simulink model "MIL_MarleyOS_Powertrain"  (R2026a)
settings: Solver=VariableStepAuto  StopTime=10
settings Model: Creator=UsuarioPC  LastModifiedBy=UsuarioPC
settings DataIOCC: ExternalInput=CommunicationDataset  LoadExternalInput=on

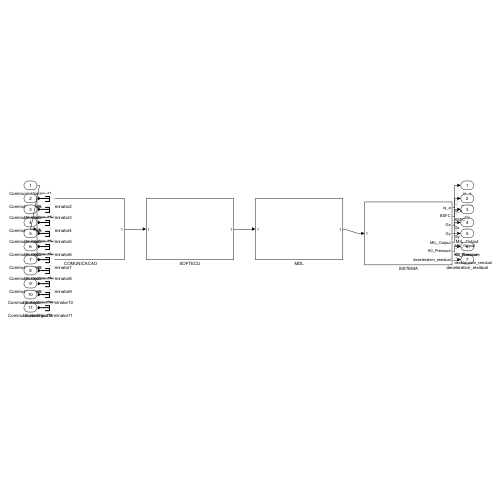
[thumbnail: Simulink's stored preview of the top-level diagram]
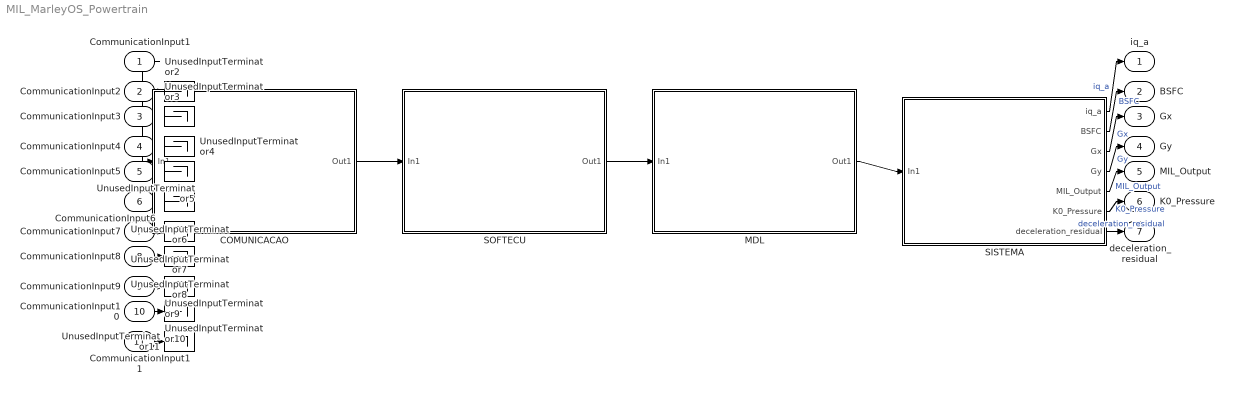
== system MIL_MarleyOS_Powertrain ==
  CommunicationInput1 : Inport
  CommunicationInput2 : Inport  Port=2
  CommunicationInput3 : Inport  Port=3
  CommunicationInput4 : Inport  Port=4
  CommunicationInput5 : Inport  Port=5
  CommunicationInput6 : Inport  Port=6
  CommunicationInput7 : Inport  Port=7
  CommunicationInput8 : Inport  Port=8
  CommunicationInput9 : Inport  Port=9
  CommunicationInput10 : Inport  Port=10
  CommunicationInput11 : Inport  Port=11
  COMUNICACAO : Subsystem
  MDL : Subsystem
  SISTEMA : Subsystem
  SOFTECU : Subsystem
  UnusedInputTerminator{2..11} (10 alike) : Terminator
  iq_a : Outport
  BSFC : Outport  Port=2
  Gx : Outport  Port=3
  Gy : Outport  Port=4
  MIL_Output : Outport  Port=5
  K0_Pressure : Outport  Port=6
  deceleration_residual : Outport  Port=7
  wires:
  CommunicationInput1/1 -> COMUNICACAO/1(In1)
  CommunicationInput2/1 -> UnusedInputTerminator2/1
  CommunicationInput3/1 -> UnusedInputTerminator3/1
  CommunicationInput4/1 -> UnusedInputTerminator4/1
  CommunicationInput5/1 -> UnusedInputTerminator5/1
  CommunicationInput6/1 -> UnusedInputTerminator6/1
  CommunicationInput7/1 -> UnusedInputTerminator7/1
  CommunicationInput8/1 -> UnusedInputTerminator8/1
  CommunicationInput9/1 -> UnusedInputTerminator9/1
  CommunicationInput10/1 -> UnusedInputTerminator10/1
  CommunicationInput11/1 -> UnusedInputTerminator11/1
  COMUNICACAO/1(Out1) -> SOFTECU/1(In1)
  SOFTECU/1(Out1) -> MDL/1(In1)
  MDL/1(Out1) -> SISTEMA/1(In1)
  SISTEMA/1(iq_a) -> iq_a/1  "iq_a"
  SISTEMA/2(BSFC) -> BSFC/1  "BSFC"
  SISTEMA/3(Gx) -> Gx/1  "Gx"
  SISTEMA/4(Gy) -> Gy/1  "Gy"
  SISTEMA/5(MIL_Output) -> MIL_Output/1  "MIL_Output"
  SISTEMA/6(K0_Pressure) -> K0_Pressure/1  "K0_Pressure"
  SISTEMA/7(deceleration_residual) -> deceleration_residual/1  "deceleration_residual"

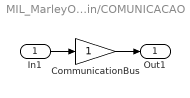
== system MIL_MarleyOS_Powertrain/COMUNICACAO ==
  In1 : Inport
  CommunicationBus : Gain
  Out1 : Outport
  wires:
  In1/1 -> CommunicationBus/1
  CommunicationBus/1 -> Out1/1

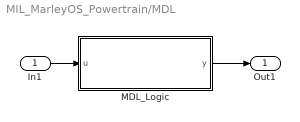
== system MIL_MarleyOS_Powertrain/MDL ==
  In1 : Inport
  MDL_Logic : MATLAB Function  TreatAsAtomicUnit=on
  Out1 : Outport
  wires:
  In1/1 -> MDL_Logic/1(u)
  MDL_Logic/1(y) -> Out1/1

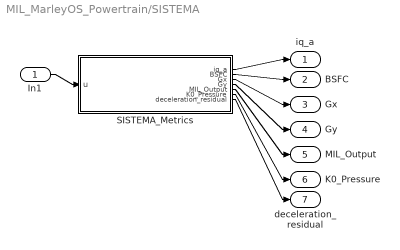
== system MIL_MarleyOS_Powertrain/SISTEMA ==
  In1 : Inport
  SISTEMA_Metrics : MATLAB Function  TreatAsAtomicUnit=on
  iq_a : Outport
  BSFC : Outport  Port=2
  Gx : Outport  Port=3
  Gy : Outport  Port=4
  MIL_Output : Outport  Port=5
  K0_Pressure : Outport  Port=6
  deceleration_residual : Outport  Port=7
  wires:
  SISTEMA_Metrics/1(iq_a) -> iq_a/1
  SISTEMA_Metrics/2(BSFC) -> BSFC/1
  SISTEMA_Metrics/3(Gx) -> Gx/1
  SISTEMA_Metrics/4(Gy) -> Gy/1
  SISTEMA_Metrics/5(MIL_Output) -> MIL_Output/1
  SISTEMA_Metrics/6(K0_Pressure) -> K0_Pressure/1
  SISTEMA_Metrics/7(deceleration_residual) -> deceleration_residual/1
  In1/1 -> SISTEMA_Metrics/1(u)

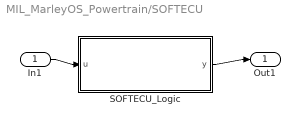
== system MIL_MarleyOS_Powertrain/SOFTECU ==
  In1 : Inport
  SOFTECU_Logic : MATLAB Function  TreatAsAtomicUnit=on
  Out1 : Outport
  wires:
  In1/1 -> SOFTECU_Logic/1(u)
  SOFTECU_Logic/1(y) -> Out1/1

== matlab function MIL_MarleyOS_Powertrain/MDL/MDL_Logic ==
  data: u input; y output
function y = mdl_logic(u)                                                         
                                                                                 % PMSM torque with flux-weakening derate and simplified vehicle inertial dynamics.
                                                                                 y = zeros(8,1,'double');                                                          
                                                                                 p = 4; lambda_pm = 0.08; J = 120;                                                 
                                                                                 iq = double(u(1));                                                                
                                                                                 vehicleSpeed = max(0, double(u(5)));                                              
                                                                                 engineRpm = vehicleSpeed * 42;                                                    
                                                                                 derate = flux_weakening_derate(engineRpm, abs(iq));                               
                                                                                 lambda_eff = lambda_pm * derate;                                                  
                                                                                 Tem = 1.5 * p * lambda_eff * iq;                                                  
                                                                                 accel = Tem / J;                                                                  
                                                                                 gx = accel / 9.81; gy = 0;                                                        
                                                                                 bsfc = 250 + abs(Tem) * 0.05;                                                     
                                                                                 y = [iq; bsfc; gx; gy; Tem; vehicleSpeed; engineRpm; double(u(2))];               
                                                                                 end                                                                               
                                                                                                                                                                   
                                                                                 function factor = flux_weakening_derate(speedRpm, iqAbs)                          
                                                                                 % 2D saturation table: PMSM effective flux derate vs speed and i_q.               
                                                                                 speedBp = [0 3000 5000 7000 9000];                                                
                                                                                 iqBp = [0 100 200 300 400];                                                       
                                                                                 derateTable = [1.00 1.00 1.00 1.00 1.00; ...                                      
                                                                                          1.00 1.00 1.00 1.00 1.00; ...                                            
                                                                                          1.00 0.97 0.93 0.88 0.82; ...                                            
                                                                                          0.95 0.90 0.83 0.75 0.65; ...                                            
                                                                                          0.85 0.78 0.68 0.55 0.40];                                               
                                                                                 s = min(max(speedRpm, speedBp(1)), speedBp(end));                                 
                                                                                 q = min(max(iqAbs, iqBp(1)), iqBp(end));                                          
                                                                                 si = 1;                                                                           
                                                                                 if s >= speedBp(4), si = 4;                                                       
                                                                                 elseif s >= speedBp(3), si = 3;                                                   
                                                                                 elseif s >= speedBp(2), si = 2;                                                   
                                                                                 else, si = 1;                                                                     
                                                                                 end                                                                               
                                                                                 qi = 1;                                                                           
                                                                                 if q >= iqBp(4), qi = 4;                                                          
                                                                                 elseif q >= iqBp(3), qi = 3;                                                      
                                                                                 elseif q >= iqBp(2), qi = 2;                                                      
                                                                                 else, qi = 1;                                                                     
                                                                                 end                                                                               
                                                                                 sFrac = (s - speedBp(si)) / (speedBp(si + 1) - speedBp(si));                      
                                                                                 qFrac = (q - iqBp(qi)) / (iqBp(qi + 1) - iqBp(qi));                               
                                                                                 topLeft = derateTable(si, qi); topRight = derateTable(si, qi + 1);                
                                                                                 botLeft = derateTable(si + 1, qi); botRight = derateTable(si + 1, qi + 1);        
                                                                                 top = topLeft + (topRight - topLeft) * qFrac;                                     
                                                                                 bot = botLeft + (botRight - botLeft) * qFrac;                                     
                                                                                 factor = top + (bot - top) * sFrac;                                               
                                                                                 end

== matlab function MIL_MarleyOS_Powertrain/SOFTECU/SOFTECU_Logic ==
  data: u input; y output; Calib_K0_PressureMax parameter double
function y = sofecu_logic(u, Calib_K0_PressureMax)                                                  
                                                                             % K0: OPEN -> SYNC -> SLIP -> LOCKED, pressure limited to 18 bar.             
                                                                             y = zeros(5,1,'double');                                                      
                                                                             speed = double(u(1));                                                         
                                                                             deltaOmega = abs(speed * 0.1);                                                
                                                                             if deltaOmega > 20                                                            
                                                                                 k0State = 0; k0Pressure = 0;                                              
                                                                             elseif deltaOmega > 8                                                         
                                                                                 k0State = 1; k0Pressure = 6;                                              
                                                                             elseif deltaOmega > 1                                                         
                                                                                 k0State = 2; k0Pressure = min(Calib_K0_PressureMax, 6 + (8-deltaOmega)*2);
                                                                             else                                                                          
                                                                                 k0State = 3; k0Pressure = Calib_K0_PressureMax;                           
                                                                             end                                                                           
                                                                             gear = min(6, max(1, floor(abs(speed)/10)+1));                                
                                                                             clutch = 1 + mod(gear, 2);                                                    
                                                                             iq = max(-200, min(200, speed * 0.5));                                        
                                                                             y = [iq; k0Pressure; k0State; clutch; gear];                                  
                                                                             end

== matlab function MIL_MarleyOS_Powertrain/SISTEMA/SISTEMA_Metrics ==
  data: u input; iq_a output; BSFC output; Gx output; Gy output; MIL_Output output; K0_Pressure output; deceleration_residual output
function [iq_a, BSFC, Gx, Gy, MIL_Output, K0_Pressure, deceleration_residual] = sistema_metrics(u)
                                                                                                 iq_a = u(1); BSFC = u(2); Gx = u(3); Gy = u(4);                                                   
                                                                                                 MIL_Output = u(5); K0_Pressure = u(8); deceleration_residual = abs(u(3));                         
                                                                                                 end
